simulink model "FKtest3"  (Simulink 6.6)
settings: Solver=ode4  StartTime=0.0  StopTime=400  FixedStep=0.05  RelTol=1e-3
undefined symbols (not defined in the file or in its folder): vessel
libraries: marine_gnc x7, simulink x2
(part 2 of 2)

== system FKtest3/Wave loads for heading2/Wave component loop/[-pi pi] to [0 2pi] ==
  note: x
  x [-pi pi] : Inport
  Constant : Constant  Value=2*pi
  Constant1 : Constant  Value=0
  Sign : Signum
  Sum : Sum  Inputs=|++  SaturateOnIntegerOverflow=on
  Switch : Switch
  0<y<2pi : Outport
  wires:
  x [-pi pi]/1 -> Sign/1, Sum/2
  Switch/1 -> Sum/1
  Sum/1 -> 0<y<2pi/1
  Sign/1 -> Switch/2
  Constant/1 -> Switch/3
  Constant1/1 -> Switch/1

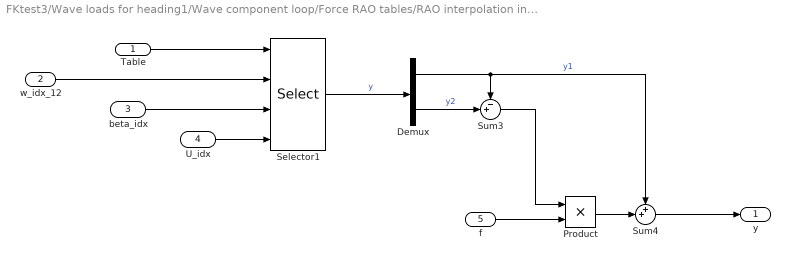
== system FKtest3/Wave loads for heading1/Wave component loop/Force RAO tables/RAO interpolation in frequency1 ==
  Table : Inport
  w_idx_12 : Inport  Port=2
  beta_idx : Inport  Port=3
  U_idx : Inport  Port=4
  f : Inport  Port=5
  Demux : Demux  Outputs=2
  Product : Product  RndMeth=Zero
  Selector1 : Selector  NumberOfDimensions=3  IndexOptions=Index vector (port),Index vector (port),Index vector (port)  Indices=[1 3],1,1  OutputSizes=1,1,1
  Sum3 : Sum  Inputs=-+|
  Sum4 : Sum  Inputs=++|
  y : Outport
  wires:
  Table/1 -> Selector1/1
  beta_idx/1 -> Selector1/3
  U_idx/1 -> Selector1/4
  Sum4/1 -> y/1
  Sum3/1 -> Product/1
  Product/1 -> Sum4/2
  Demux/1 -> Sum4/1, Sum3/1  "y1"
  Demux/2 -> Sum3/2  "y2"
  Selector1/1 -> Demux/1  "y"
  w_idx_12/1 -> Selector1/2
  f/1 -> Product/2

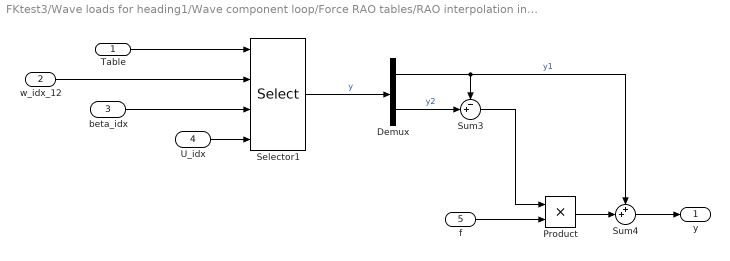
== system FKtest3/Wave loads for heading1/Wave component loop/Force RAO tables/RAO interpolation in frequency10 ==
  Table : Inport
  w_idx_12 : Inport  Port=2
  beta_idx : Inport  Port=3
  U_idx : Inport  Port=4
  f : Inport  Port=5
  Demux : Demux  Outputs=2
  Product : Product  RndMeth=Zero
  Selector1 : Selector  NumberOfDimensions=3  IndexOptions=Index vector (port),Index vector (port),Index vector (port)  Indices=[1 3],1,1  OutputSizes=1,1,1
  Sum3 : Sum  Inputs=-+|
  Sum4 : Sum  Inputs=++|
  y : Outport
  wires:
  Table/1 -> Selector1/1
  beta_idx/1 -> Selector1/3
  U_idx/1 -> Selector1/4
  Sum4/1 -> y/1
  Sum3/1 -> Product/1
  Product/1 -> Sum4/2
  Demux/1 -> Sum4/1, Sum3/1  "y1"
  Demux/2 -> Sum3/2  "y2"
  Selector1/1 -> Demux/1  "y"
  w_idx_12/1 -> Selector1/2
  f/1 -> Product/2

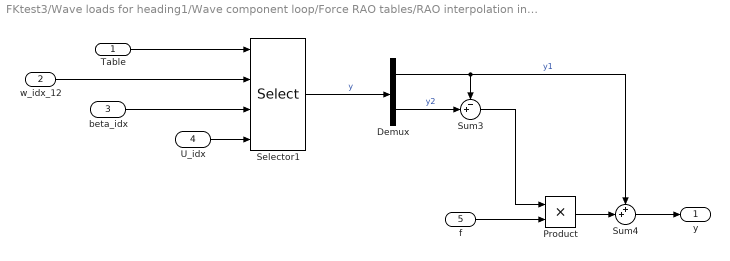
== system FKtest3/Wave loads for heading1/Wave component loop/Force RAO tables/RAO interpolation in frequency11 ==
  Table : Inport
  w_idx_12 : Inport  Port=2
  beta_idx : Inport  Port=3
  U_idx : Inport  Port=4
  f : Inport  Port=5
  Demux : Demux  Outputs=2
  Product : Product  RndMeth=Zero
  Selector1 : Selector  NumberOfDimensions=3  IndexOptions=Index vector (port),Index vector (port),Index vector (port)  Indices=[1 3],1,1  OutputSizes=1,1,1
  Sum3 : Sum  Inputs=-+|
  Sum4 : Sum  Inputs=++|
  y : Outport
  wires:
  Table/1 -> Selector1/1
  beta_idx/1 -> Selector1/3
  U_idx/1 -> Selector1/4
  Sum4/1 -> y/1
  Sum3/1 -> Product/1
  Product/1 -> Sum4/2
  Demux/1 -> Sum4/1, Sum3/1  "y1"
  Demux/2 -> Sum3/2  "y2"
  Selector1/1 -> Demux/1  "y"
  w_idx_12/1 -> Selector1/2
  f/1 -> Product/2

== system FKtest3/Wave loads for heading1/Wave component loop/Force RAO tables/RAO interpolation in frequency12 ==
  Table : Inport
  w_idx_12 : Inport  Port=2
  beta_idx : Inport  Port=3
  U_idx : Inport  Port=4
  f : Inport  Port=5
  Demux : Demux  Outputs=2
  Product : Product  RndMeth=Zero
  Selector1 : Selector  NumberOfDimensions=3  IndexOptions=Index vector (port),Index vector (port),Index vector (port)  Indices=[1 3],1,1  OutputSizes=1,1,1
  Sum3 : Sum  Inputs=-+|
  Sum4 : Sum  Inputs=++|
  y : Outport
  wires:
  Table/1 -> Selector1/1
  beta_idx/1 -> Selector1/3
  U_idx/1 -> Selector1/4
  Sum4/1 -> y/1
  Sum3/1 -> Product/1
  Product/1 -> Sum4/2
  Demux/1 -> Sum4/1, Sum3/1  "y1"
  Demux/2 -> Sum3/2  "y2"
  Selector1/1 -> Demux/1  "y"
  w_idx_12/1 -> Selector1/2
  f/1 -> Product/2

== system FKtest3/Wave loads for heading1/Wave component loop/Force RAO tables/RAO interpolation in frequency2 ==
  Table : Inport
  w_idx_12 : Inport  Port=2
  beta_idx : Inport  Port=3
  U_idx : Inport  Port=4
  f : Inport  Port=5
  Demux : Demux  Outputs=2
  Product : Product  RndMeth=Zero
  Selector1 : Selector  NumberOfDimensions=3  IndexOptions=Index vector (port),Index vector (port),Index vector (port)  Indices=[1 3],1,1  OutputSizes=1,1,1
  Sum3 : Sum  Inputs=-+|
  Sum4 : Sum  Inputs=++|
  y : Outport
  wires:
  Table/1 -> Selector1/1
  beta_idx/1 -> Selector1/3
  U_idx/1 -> Selector1/4
  Sum4/1 -> y/1
  Sum3/1 -> Product/1
  Product/1 -> Sum4/2
  Demux/1 -> Sum4/1, Sum3/1  "y1"
  Demux/2 -> Sum3/2  "y2"
  Selector1/1 -> Demux/1  "y"
  w_idx_12/1 -> Selector1/2
  f/1 -> Product/2

== system FKtest3/Wave loads for heading1/Wave component loop/Force RAO tables/RAO interpolation in frequency3 ==
  Table : Inport
  w_idx_12 : Inport  Port=2
  beta_idx : Inport  Port=3
  U_idx : Inport  Port=4
  f : Inport  Port=5
  Demux : Demux  Outputs=2
  Product : Product  RndMeth=Zero
  Selector1 : Selector  NumberOfDimensions=3  IndexOptions=Index vector (port),Index vector (port),Index vector (port)  Indices=[1 3],1,1  OutputSizes=1,1,1
  Sum3 : Sum  Inputs=-+|
  Sum4 : Sum  Inputs=++|
  y : Outport
  wires:
  Table/1 -> Selector1/1
  beta_idx/1 -> Selector1/3
  U_idx/1 -> Selector1/4
  Sum4/1 -> y/1
  Sum3/1 -> Product/1
  Product/1 -> Sum4/2
  Demux/1 -> Sum4/1, Sum3/1  "y1"
  Demux/2 -> Sum3/2  "y2"
  Selector1/1 -> Demux/1  "y"
  w_idx_12/1 -> Selector1/2
  f/1 -> Product/2

== system FKtest3/Wave loads for heading1/Wave component loop/Force RAO tables/RAO interpolation in frequency4 ==
  Table : Inport
  w_idx_12 : Inport  Port=2
  beta_idx : Inport  Port=3
  U_idx : Inport  Port=4
  f : Inport  Port=5
  Demux : Demux  Outputs=2
  Product : Product  RndMeth=Zero
  Selector1 : Selector  NumberOfDimensions=3  IndexOptions=Index vector (port),Index vector (port),Index vector (port)  Indices=[1 3],1,1  OutputSizes=1,1,1
  Sum3 : Sum  Inputs=-+|
  Sum4 : Sum  Inputs=++|
  y : Outport
  wires:
  Table/1 -> Selector1/1
  beta_idx/1 -> Selector1/3
  U_idx/1 -> Selector1/4
  Sum4/1 -> y/1
  Sum3/1 -> Product/1
  Product/1 -> Sum4/2
  Demux/1 -> Sum4/1, Sum3/1  "y1"
  Demux/2 -> Sum3/2  "y2"
  Selector1/1 -> Demux/1  "y"
  w_idx_12/1 -> Selector1/2
  f/1 -> Product/2

== system FKtest3/Wave loads for heading1/Wave component loop/Force RAO tables/RAO interpolation in frequency5 ==
  Table : Inport
  w_idx_12 : Inport  Port=2
  beta_idx : Inport  Port=3
  U_idx : Inport  Port=4
  f : Inport  Port=5
  Demux : Demux  Outputs=2
  Product : Product  RndMeth=Zero
  Selector1 : Selector  NumberOfDimensions=3  IndexOptions=Index vector (port),Index vector (port),Index vector (port)  Indices=[1 3],1,1  OutputSizes=1,1,1
  Sum3 : Sum  Inputs=-+|
  Sum4 : Sum  Inputs=++|
  y : Outport
  wires:
  Table/1 -> Selector1/1
  beta_idx/1 -> Selector1/3
  U_idx/1 -> Selector1/4
  Sum4/1 -> y/1
  Sum3/1 -> Product/1
  Product/1 -> Sum4/2
  Demux/1 -> Sum4/1, Sum3/1  "y1"
  Demux/2 -> Sum3/2  "y2"
  Selector1/1 -> Demux/1  "y"
  w_idx_12/1 -> Selector1/2
  f/1 -> Product/2

== system FKtest3/Wave loads for heading1/Wave component loop/Force RAO tables/RAO interpolation in frequency6 ==
  Table : Inport
  w_idx_12 : Inport  Port=2
  beta_idx : Inport  Port=3
  U_idx : Inport  Port=4
  f : Inport  Port=5
  Demux : Demux  Outputs=2
  Product : Product  RndMeth=Zero
  Selector1 : Selector  NumberOfDimensions=3  IndexOptions=Index vector (port),Index vector (port),Index vector (port)  Indices=[1 3],1,1  OutputSizes=1,1,1
  Sum3 : Sum  Inputs=-+|
  Sum4 : Sum  Inputs=++|
  y : Outport
  wires:
  Table/1 -> Selector1/1
  beta_idx/1 -> Selector1/3
  U_idx/1 -> Selector1/4
  Sum4/1 -> y/1
  Sum3/1 -> Product/1
  Product/1 -> Sum4/2
  Demux/1 -> Sum4/1, Sum3/1  "y1"
  Demux/2 -> Sum3/2  "y2"
  Selector1/1 -> Demux/1  "y"
  w_idx_12/1 -> Selector1/2
  f/1 -> Product/2

== system FKtest3/Wave loads for heading1/Wave component loop/Force RAO tables/RAO interpolation in frequency7 ==
  Table : Inport
  w_idx_12 : Inport  Port=2
  beta_idx : Inport  Port=3
  U_idx : Inport  Port=4
  f : Inport  Port=5
  Demux : Demux  Outputs=2
  Product : Product  RndMeth=Zero
  Selector1 : Selector  NumberOfDimensions=3  IndexOptions=Index vector (port),Index vector (port),Index vector (port)  Indices=[1 3],1,1  OutputSizes=1,1,1
  Sum3 : Sum  Inputs=-+|
  Sum4 : Sum  Inputs=++|
  y : Outport
  wires:
  Table/1 -> Selector1/1
  beta_idx/1 -> Selector1/3
  U_idx/1 -> Selector1/4
  Sum4/1 -> y/1
  Sum3/1 -> Product/1
  Product/1 -> Sum4/2
  Demux/1 -> Sum4/1, Sum3/1  "y1"
  Demux/2 -> Sum3/2  "y2"
  Selector1/1 -> Demux/1  "y"
  w_idx_12/1 -> Selector1/2
  f/1 -> Product/2

== system FKtest3/Wave loads for heading1/Wave component loop/Force RAO tables/RAO interpolation in frequency8 ==
  Table : Inport
  w_idx_12 : Inport  Port=2
  beta_idx : Inport  Port=3
  U_idx : Inport  Port=4
  f : Inport  Port=5
  Demux : Demux  Outputs=2
  Product : Product  RndMeth=Zero
  Selector1 : Selector  NumberOfDimensions=3  IndexOptions=Index vector (port),Index vector (port),Index vector (port)  Indices=[1 3],1,1  OutputSizes=1,1,1
  Sum3 : Sum  Inputs=-+|
  Sum4 : Sum  Inputs=++|
  y : Outport
  wires:
  Table/1 -> Selector1/1
  beta_idx/1 -> Selector1/3
  U_idx/1 -> Selector1/4
  Sum4/1 -> y/1
  Sum3/1 -> Product/1
  Product/1 -> Sum4/2
  Demux/1 -> Sum4/1, Sum3/1  "y1"
  Demux/2 -> Sum3/2  "y2"
  Selector1/1 -> Demux/1  "y"
  w_idx_12/1 -> Selector1/2
  f/1 -> Product/2

== system FKtest3/Wave loads for heading1/Wave component loop/Force RAO tables/RAO interpolation in frequency9 ==
  Table : Inport
  w_idx_12 : Inport  Port=2
  beta_idx : Inport  Port=3
  U_idx : Inport  Port=4
  f : Inport  Port=5
  Demux : Demux  Outputs=2
  Product : Product  RndMeth=Zero
  Selector1 : Selector  NumberOfDimensions=3  IndexOptions=Index vector (port),Index vector (port),Index vector (port)  Indices=[1 3],1,1  OutputSizes=1,1,1
  Sum3 : Sum  Inputs=-+|
  Sum4 : Sum  Inputs=++|
  y : Outport
  wires:
  Table/1 -> Selector1/1
  beta_idx/1 -> Selector1/3
  U_idx/1 -> Selector1/4
  Sum4/1 -> y/1
  Sum3/1 -> Product/1
  Product/1 -> Sum4/2
  Demux/1 -> Sum4/1, Sum3/1  "y1"
  Demux/2 -> Sum3/2  "y2"
  Selector1/1 -> Demux/1  "y"
  w_idx_12/1 -> Selector1/2
  f/1 -> Product/2

== system FKtest3/Wave loads for heading1/Wave component loop/WD RAO tables/RAO interpolation in frequency1 ==
  Table : Inport
  w_idx_12 : Inport  Port=2
  beta_idx : Inport  Port=3
  U_idx : Inport  Port=4
  f : Inport  Port=5
  Demux : Demux  Outputs=2
  Product : Product  RndMeth=Zero
  Selector1 : Selector  NumberOfDimensions=3  IndexOptions=Index vector (port),Index vector (port),Index vector (port)  Indices=[1 3],1,1  OutputSizes=1,1,1
  Sum3 : Sum  Inputs=-+|
  Sum4 : Sum  Inputs=++|
  y : Outport
  wires:
  Table/1 -> Selector1/1
  beta_idx/1 -> Selector1/3
  U_idx/1 -> Selector1/4
  Sum4/1 -> y/1
  Sum3/1 -> Product/1
  Product/1 -> Sum4/2
  Demux/1 -> Sum4/1, Sum3/1  "y1"
  Demux/2 -> Sum3/2  "y2"
  Selector1/1 -> Demux/1  "y"
  w_idx_12/1 -> Selector1/2
  f/1 -> Product/2

== system FKtest3/Wave loads for heading1/Wave component loop/WD RAO tables/RAO interpolation in frequency2 ==
  Table : Inport
  w_idx_12 : Inport  Port=2
  beta_idx : Inport  Port=3
  U_idx : Inport  Port=4
  f : Inport  Port=5
  Demux : Demux  Outputs=2
  Product : Product  RndMeth=Zero
  Selector1 : Selector  NumberOfDimensions=3  IndexOptions=Index vector (port),Index vector (port),Index vector (port)  Indices=[1 3],1,1  OutputSizes=1,1,1
  Sum3 : Sum  Inputs=-+|
  Sum4 : Sum  Inputs=++|
  y : Outport
  wires:
  Table/1 -> Selector1/1
  beta_idx/1 -> Selector1/3
  U_idx/1 -> Selector1/4
  Sum4/1 -> y/1
  Sum3/1 -> Product/1
  Product/1 -> Sum4/2
  Demux/1 -> Sum4/1, Sum3/1  "y1"
  Demux/2 -> Sum3/2  "y2"
  Selector1/1 -> Demux/1  "y"
  w_idx_12/1 -> Selector1/2
  f/1 -> Product/2

== system FKtest3/Wave loads for heading1/Wave component loop/WD RAO tables/RAO interpolation in frequency3 ==
  Table : Inport
  w_idx_12 : Inport  Port=2
  beta_idx : Inport  Port=3
  U_idx : Inport  Port=4
  f : Inport  Port=5
  Demux : Demux  Outputs=2
  Product : Product  RndMeth=Zero
  Selector1 : Selector  NumberOfDimensions=3  IndexOptions=Index vector (port),Index vector (port),Index vector (port)  Indices=[1 3],1,1  OutputSizes=1,1,1
  Sum3 : Sum  Inputs=-+|
  Sum4 : Sum  Inputs=++|
  y : Outport
  wires:
  Table/1 -> Selector1/1
  beta_idx/1 -> Selector1/3
  U_idx/1 -> Selector1/4
  Sum4/1 -> y/1
  Sum3/1 -> Product/1
  Product/1 -> Sum4/2
  Demux/1 -> Sum4/1, Sum3/1  "y1"
  Demux/2 -> Sum3/2  "y2"
  Selector1/1 -> Demux/1  "y"
  w_idx_12/1 -> Selector1/2
  f/1 -> Product/2

== system FKtest3/Wave loads for heading2/Wave component loop/Force RAO tables/RAO interpolation in frequency1 ==
  Table : Inport
  w_idx_12 : Inport  Port=2
  beta_idx : Inport  Port=3
  U_idx : Inport  Port=4
  f : Inport  Port=5
  Demux : Demux  Outputs=2
  Product : Product  RndMeth=Zero
  Selector1 : Selector  NumberOfDimensions=3  IndexOptions=Index vector (port),Index vector (port),Index vector (port)  Indices=[1 3],1,1  OutputSizes=1,1,1
  Sum3 : Sum  Inputs=-+|
  Sum4 : Sum  Inputs=++|
  y : Outport
  wires:
  Table/1 -> Selector1/1
  beta_idx/1 -> Selector1/3
  U_idx/1 -> Selector1/4
  Sum4/1 -> y/1
  Sum3/1 -> Product/1
  Product/1 -> Sum4/2
  Demux/1 -> Sum4/1, Sum3/1  "y1"
  Demux/2 -> Sum3/2  "y2"
  Selector1/1 -> Demux/1  "y"
  w_idx_12/1 -> Selector1/2
  f/1 -> Product/2

== system FKtest3/Wave loads for heading2/Wave component loop/Force RAO tables/RAO interpolation in frequency10 ==
  Table : Inport
  w_idx_12 : Inport  Port=2
  beta_idx : Inport  Port=3
  U_idx : Inport  Port=4
  f : Inport  Port=5
  Demux : Demux  Outputs=2
  Product : Product  RndMeth=Zero
  Selector1 : Selector  NumberOfDimensions=3  IndexOptions=Index vector (port),Index vector (port),Index vector (port)  Indices=[1 3],1,1  OutputSizes=1,1,1
  Sum3 : Sum  Inputs=-+|
  Sum4 : Sum  Inputs=++|
  y : Outport
  wires:
  Table/1 -> Selector1/1
  beta_idx/1 -> Selector1/3
  U_idx/1 -> Selector1/4
  Sum4/1 -> y/1
  Sum3/1 -> Product/1
  Product/1 -> Sum4/2
  Demux/1 -> Sum4/1, Sum3/1  "y1"
  Demux/2 -> Sum3/2  "y2"
  Selector1/1 -> Demux/1  "y"
  w_idx_12/1 -> Selector1/2
  f/1 -> Product/2

== system FKtest3/Wave loads for heading2/Wave component loop/Force RAO tables/RAO interpolation in frequency11 ==
  Table : Inport
  w_idx_12 : Inport  Port=2
  beta_idx : Inport  Port=3
  U_idx : Inport  Port=4
  f : Inport  Port=5
  Demux : Demux  Outputs=2
  Product : Product  RndMeth=Zero
  Selector1 : Selector  NumberOfDimensions=3  IndexOptions=Index vector (port),Index vector (port),Index vector (port)  Indices=[1 3],1,1  OutputSizes=1,1,1
  Sum3 : Sum  Inputs=-+|
  Sum4 : Sum  Inputs=++|
  y : Outport
  wires:
  Table/1 -> Selector1/1
  beta_idx/1 -> Selector1/3
  U_idx/1 -> Selector1/4
  Sum4/1 -> y/1
  Sum3/1 -> Product/1
  Product/1 -> Sum4/2
  Demux/1 -> Sum4/1, Sum3/1  "y1"
  Demux/2 -> Sum3/2  "y2"
  Selector1/1 -> Demux/1  "y"
  w_idx_12/1 -> Selector1/2
  f/1 -> Product/2

== system FKtest3/Wave loads for heading2/Wave component loop/Force RAO tables/RAO interpolation in frequency12 ==
  Table : Inport
  w_idx_12 : Inport  Port=2
  beta_idx : Inport  Port=3
  U_idx : Inport  Port=4
  f : Inport  Port=5
  Demux : Demux  Outputs=2
  Product : Product  RndMeth=Zero
  Selector1 : Selector  NumberOfDimensions=3  IndexOptions=Index vector (port),Index vector (port),Index vector (port)  Indices=[1 3],1,1  OutputSizes=1,1,1
  Sum3 : Sum  Inputs=-+|
  Sum4 : Sum  Inputs=++|
  y : Outport
  wires:
  Table/1 -> Selector1/1
  beta_idx/1 -> Selector1/3
  U_idx/1 -> Selector1/4
  Sum4/1 -> y/1
  Sum3/1 -> Product/1
  Product/1 -> Sum4/2
  Demux/1 -> Sum4/1, Sum3/1  "y1"
  Demux/2 -> Sum3/2  "y2"
  Selector1/1 -> Demux/1  "y"
  w_idx_12/1 -> Selector1/2
  f/1 -> Product/2

== system FKtest3/Wave loads for heading2/Wave component loop/Force RAO tables/RAO interpolation in frequency2 ==
  Table : Inport
  w_idx_12 : Inport  Port=2
  beta_idx : Inport  Port=3
  U_idx : Inport  Port=4
  f : Inport  Port=5
  Demux : Demux  Outputs=2
  Product : Product  RndMeth=Zero
  Selector1 : Selector  NumberOfDimensions=3  IndexOptions=Index vector (port),Index vector (port),Index vector (port)  Indices=[1 3],1,1  OutputSizes=1,1,1
  Sum3 : Sum  Inputs=-+|
  Sum4 : Sum  Inputs=++|
  y : Outport
  wires:
  Table/1 -> Selector1/1
  beta_idx/1 -> Selector1/3
  U_idx/1 -> Selector1/4
  Sum4/1 -> y/1
  Sum3/1 -> Product/1
  Product/1 -> Sum4/2
  Demux/1 -> Sum4/1, Sum3/1  "y1"
  Demux/2 -> Sum3/2  "y2"
  Selector1/1 -> Demux/1  "y"
  w_idx_12/1 -> Selector1/2
  f/1 -> Product/2

== system FKtest3/Wave loads for heading2/Wave component loop/Force RAO tables/RAO interpolation in frequency3 ==
  Table : Inport
  w_idx_12 : Inport  Port=2
  beta_idx : Inport  Port=3
  U_idx : Inport  Port=4
  f : Inport  Port=5
  Demux : Demux  Outputs=2
  Product : Product  RndMeth=Zero
  Selector1 : Selector  NumberOfDimensions=3  IndexOptions=Index vector (port),Index vector (port),Index vector (port)  Indices=[1 3],1,1  OutputSizes=1,1,1
  Sum3 : Sum  Inputs=-+|
  Sum4 : Sum  Inputs=++|
  y : Outport
  wires:
  Table/1 -> Selector1/1
  beta_idx/1 -> Selector1/3
  U_idx/1 -> Selector1/4
  Sum4/1 -> y/1
  Sum3/1 -> Product/1
  Product/1 -> Sum4/2
  Demux/1 -> Sum4/1, Sum3/1  "y1"
  Demux/2 -> Sum3/2  "y2"
  Selector1/1 -> Demux/1  "y"
  w_idx_12/1 -> Selector1/2
  f/1 -> Product/2

== system FKtest3/Wave loads for heading2/Wave component loop/Force RAO tables/RAO interpolation in frequency4 ==
  Table : Inport
  w_idx_12 : Inport  Port=2
  beta_idx : Inport  Port=3
  U_idx : Inport  Port=4
  f : Inport  Port=5
  Demux : Demux  Outputs=2
  Product : Product  RndMeth=Zero
  Selector1 : Selector  NumberOfDimensions=3  IndexOptions=Index vector (port),Index vector (port),Index vector (port)  Indices=[1 3],1,1  OutputSizes=1,1,1
  Sum3 : Sum  Inputs=-+|
  Sum4 : Sum  Inputs=++|
  y : Outport
  wires:
  Table/1 -> Selector1/1
  beta_idx/1 -> Selector1/3
  U_idx/1 -> Selector1/4
  Sum4/1 -> y/1
  Sum3/1 -> Product/1
  Product/1 -> Sum4/2
  Demux/1 -> Sum4/1, Sum3/1  "y1"
  Demux/2 -> Sum3/2  "y2"
  Selector1/1 -> Demux/1  "y"
  w_idx_12/1 -> Selector1/2
  f/1 -> Product/2

== system FKtest3/Wave loads for heading2/Wave component loop/Force RAO tables/RAO interpolation in frequency5 ==
  Table : Inport
  w_idx_12 : Inport  Port=2
  beta_idx : Inport  Port=3
  U_idx : Inport  Port=4
  f : Inport  Port=5
  Demux : Demux  Outputs=2
  Product : Product  RndMeth=Zero
  Selector1 : Selector  NumberOfDimensions=3  IndexOptions=Index vector (port),Index vector (port),Index vector (port)  Indices=[1 3],1,1  OutputSizes=1,1,1
  Sum3 : Sum  Inputs=-+|
  Sum4 : Sum  Inputs=++|
  y : Outport
  wires:
  Table/1 -> Selector1/1
  beta_idx/1 -> Selector1/3
  U_idx/1 -> Selector1/4
  Sum4/1 -> y/1
  Sum3/1 -> Product/1
  Product/1 -> Sum4/2
  Demux/1 -> Sum4/1, Sum3/1  "y1"
  Demux/2 -> Sum3/2  "y2"
  Selector1/1 -> Demux/1  "y"
  w_idx_12/1 -> Selector1/2
  f/1 -> Product/2

== system FKtest3/Wave loads for heading2/Wave component loop/Force RAO tables/RAO interpolation in frequency6 ==
  Table : Inport
  w_idx_12 : Inport  Port=2
  beta_idx : Inport  Port=3
  U_idx : Inport  Port=4
  f : Inport  Port=5
  Demux : Demux  Outputs=2
  Product : Product  RndMeth=Zero
  Selector1 : Selector  NumberOfDimensions=3  IndexOptions=Index vector (port),Index vector (port),Index vector (port)  Indices=[1 3],1,1  OutputSizes=1,1,1
  Sum3 : Sum  Inputs=-+|
  Sum4 : Sum  Inputs=++|
  y : Outport
  wires:
  Table/1 -> Selector1/1
  beta_idx/1 -> Selector1/3
  U_idx/1 -> Selector1/4
  Sum4/1 -> y/1
  Sum3/1 -> Product/1
  Product/1 -> Sum4/2
  Demux/1 -> Sum4/1, Sum3/1  "y1"
  Demux/2 -> Sum3/2  "y2"
  Selector1/1 -> Demux/1  "y"
  w_idx_12/1 -> Selector1/2
  f/1 -> Product/2

== system FKtest3/Wave loads for heading2/Wave component loop/Force RAO tables/RAO interpolation in frequency7 ==
  Table : Inport
  w_idx_12 : Inport  Port=2
  beta_idx : Inport  Port=3
  U_idx : Inport  Port=4
  f : Inport  Port=5
  Demux : Demux  Outputs=2
  Product : Product  RndMeth=Zero
  Selector1 : Selector  NumberOfDimensions=3  IndexOptions=Index vector (port),Index vector (port),Index vector (port)  Indices=[1 3],1,1  OutputSizes=1,1,1
  Sum3 : Sum  Inputs=-+|
  Sum4 : Sum  Inputs=++|
  y : Outport
  wires:
  Table/1 -> Selector1/1
  beta_idx/1 -> Selector1/3
  U_idx/1 -> Selector1/4
  Sum4/1 -> y/1
  Sum3/1 -> Product/1
  Product/1 -> Sum4/2
  Demux/1 -> Sum4/1, Sum3/1  "y1"
  Demux/2 -> Sum3/2  "y2"
  Selector1/1 -> Demux/1  "y"
  w_idx_12/1 -> Selector1/2
  f/1 -> Product/2

== system FKtest3/Wave loads for heading2/Wave component loop/Force RAO tables/RAO interpolation in frequency8 ==
  Table : Inport
  w_idx_12 : Inport  Port=2
  beta_idx : Inport  Port=3
  U_idx : Inport  Port=4
  f : Inport  Port=5
  Demux : Demux  Outputs=2
  Product : Product  RndMeth=Zero
  Selector1 : Selector  NumberOfDimensions=3  IndexOptions=Index vector (port),Index vector (port),Index vector (port)  Indices=[1 3],1,1  OutputSizes=1,1,1
  Sum3 : Sum  Inputs=-+|
  Sum4 : Sum  Inputs=++|
  y : Outport
  wires:
  Table/1 -> Selector1/1
  beta_idx/1 -> Selector1/3
  U_idx/1 -> Selector1/4
  Sum4/1 -> y/1
  Sum3/1 -> Product/1
  Product/1 -> Sum4/2
  Demux/1 -> Sum4/1, Sum3/1  "y1"
  Demux/2 -> Sum3/2  "y2"
  Selector1/1 -> Demux/1  "y"
  w_idx_12/1 -> Selector1/2
  f/1 -> Product/2

== system FKtest3/Wave loads for heading2/Wave component loop/Force RAO tables/RAO interpolation in frequency9 ==
  Table : Inport
  w_idx_12 : Inport  Port=2
  beta_idx : Inport  Port=3
  U_idx : Inport  Port=4
  f : Inport  Port=5
  Demux : Demux  Outputs=2
  Product : Product  RndMeth=Zero
  Selector1 : Selector  NumberOfDimensions=3  IndexOptions=Index vector (port),Index vector (port),Index vector (port)  Indices=[1 3],1,1  OutputSizes=1,1,1
  Sum3 : Sum  Inputs=-+|
  Sum4 : Sum  Inputs=++|
  y : Outport
  wires:
  Table/1 -> Selector1/1
  beta_idx/1 -> Selector1/3
  U_idx/1 -> Selector1/4
  Sum4/1 -> y/1
  Sum3/1 -> Product/1
  Product/1 -> Sum4/2
  Demux/1 -> Sum4/1, Sum3/1  "y1"
  Demux/2 -> Sum3/2  "y2"
  Selector1/1 -> Demux/1  "y"
  w_idx_12/1 -> Selector1/2
  f/1 -> Product/2

== system FKtest3/Wave loads for heading2/Wave component loop/WD RAO tables/RAO interpolation in frequency1 ==
  Table : Inport
  w_idx_12 : Inport  Port=2
  beta_idx : Inport  Port=3
  U_idx : Inport  Port=4
  f : Inport  Port=5
  Demux : Demux  Outputs=2
  Product : Product  RndMeth=Zero
  Selector1 : Selector  NumberOfDimensions=3  IndexOptions=Index vector (port),Index vector (port),Index vector (port)  Indices=[1 3],1,1  OutputSizes=1,1,1
  Sum3 : Sum  Inputs=-+|
  Sum4 : Sum  Inputs=++|
  y : Outport
  wires:
  Table/1 -> Selector1/1
  beta_idx/1 -> Selector1/3
  U_idx/1 -> Selector1/4
  Sum4/1 -> y/1
  Sum3/1 -> Product/1
  Product/1 -> Sum4/2
  Demux/1 -> Sum4/1, Sum3/1  "y1"
  Demux/2 -> Sum3/2  "y2"
  Selector1/1 -> Demux/1  "y"
  w_idx_12/1 -> Selector1/2
  f/1 -> Product/2

== system FKtest3/Wave loads for heading2/Wave component loop/WD RAO tables/RAO interpolation in frequency2 ==
  Table : Inport
  w_idx_12 : Inport  Port=2
  beta_idx : Inport  Port=3
  U_idx : Inport  Port=4
  f : Inport  Port=5
  Demux : Demux  Outputs=2
  Product : Product  RndMeth=Zero
  Selector1 : Selector  NumberOfDimensions=3  IndexOptions=Index vector (port),Index vector (port),Index vector (port)  Indices=[1 3],1,1  OutputSizes=1,1,1
  Sum3 : Sum  Inputs=-+|
  Sum4 : Sum  Inputs=++|
  y : Outport
  wires:
  Table/1 -> Selector1/1
  beta_idx/1 -> Selector1/3
  U_idx/1 -> Selector1/4
  Sum4/1 -> y/1
  Sum3/1 -> Product/1
  Product/1 -> Sum4/2
  Demux/1 -> Sum4/1, Sum3/1  "y1"
  Demux/2 -> Sum3/2  "y2"
  Selector1/1 -> Demux/1  "y"
  w_idx_12/1 -> Selector1/2
  f/1 -> Product/2

== system FKtest3/Wave loads for heading2/Wave component loop/WD RAO tables/RAO interpolation in frequency3 ==
  Table : Inport
  w_idx_12 : Inport  Port=2
  beta_idx : Inport  Port=3
  U_idx : Inport  Port=4
  f : Inport  Port=5
  Demux : Demux  Outputs=2
  Product : Product  RndMeth=Zero
  Selector1 : Selector  NumberOfDimensions=3  IndexOptions=Index vector (port),Index vector (port),Index vector (port)  Indices=[1 3],1,1  OutputSizes=1,1,1
  Sum3 : Sum  Inputs=-+|
  Sum4 : Sum  Inputs=++|
  y : Outport
  wires:
  Table/1 -> Selector1/1
  beta_idx/1 -> Selector1/3
  U_idx/1 -> Selector1/4
  Sum4/1 -> y/1
  Sum3/1 -> Product/1
  Product/1 -> Sum4/2
  Demux/1 -> Sum4/1, Sum3/1  "y1"
  Demux/2 -> Sum3/2  "y2"
  Selector1/1 -> Demux/1  "y"
  w_idx_12/1 -> Selector1/2
  f/1 -> Product/2
